simulink model "sep_step"  (R2018b)
settings: Solver=VariableStepAuto  StartTime=0.0  StopTime=100  RelTol=1e-3
settings Model: Creator=jh2044  LastModifiedBy=jh2044

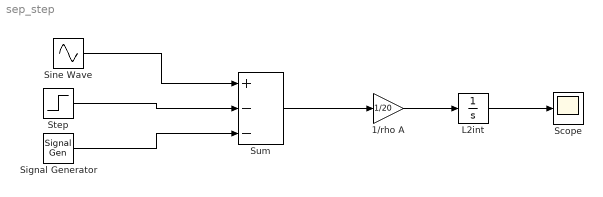
== system sep_step ==
  1/rho A : Gain  Gain=1/20
  L2int : Integrator
  Scope : Scope
  Signal Generator : SignalGenerator  WaveForm=random  Amplitude=5  Units=rad/sec
  Sine Wave : Sin  Amplitude=5  SampleTime=0
  Step : Step  SampleTime=0
  Sum : Sum  Inputs=+--
  wires:
  L2int/1 -> Scope/1
  Sum/1 -> 1/rho A/1
  1/rho A/1 -> L2int/1
  Sine Wave/1 -> Sum/1
  Step/1 -> Sum/2
  Signal Generator/1 -> Sum/3
